simulink library "SUB_ECU_L4_MABX_HW_Interface"  (R2018a)
settings: Solver=VariableStepAuto  StartTime=0.0  StopTime=10.0  RelTol=1e-3
PostLoadFcn:
  | , if any(exist('dsrtsu_mdlpostloadfcn', 'file') == [2, 3, 6]), try dsrtsu_mdlpostloadfcn('Execute', bdroot); catch fprintf('Error in PostLoadFcn (dsrtsu_mdlpostloadfcn) for model "%s":\n %s\n', bdroot, lasterr); end, end,
undefined symbols (not defined in the file or in its folder): CANR_PROPB_REAX_3_13_CHANNEL_APV, CANR_PROPB_REAX_4_13_CHANNEL_APV, CANR_PROPB_XPR_1_50_CHANNEL_APV, ENUM_CAN_RX_T, ENUM_CAN_TX_T, ENUM_REAX_OPERATION_MODE_T, ENUM_SIGNAL_HEALTH_T, ENUM_XBR_CONTROL_MODE_T, ENUM_XBR_EBI_MODE_T, ENUM_XBR_PASS_THROUGH_ACTIVE_T, ENUM_XBR_PRIORITY_T, ENUM_XPR_INHIBIT_PARK_MANUAL_T, ENUM_XPR_INHIBIT_UNPARK_MANUAL_T, ENUM_XPR_PARK_MANUAL_T, ENUM_XPR_UNPARK_MANUAL_T, PROPB_REAX_1_E4_DES_POS_SIG_SRC_APV, PROPB_REAX_1_E4_DESIRED_OPMODE_APV, PROPB_REAX_1_E4_DESIRED_POSITION_APV, ptc_matlab_lib
libraries: PTC_MBDS_LIB x264, rtican x172, EmE_MBD_Blockset x39, simulink x34, $bdroot x16, rti1401lib_dio_type4 x8, simulink_need_slupdate x7, dsa_tcpip_lib x4, rti1401lib_adc_type4 x3, rtmapslib x3, rtitasklib x3
(part 33 of 51)

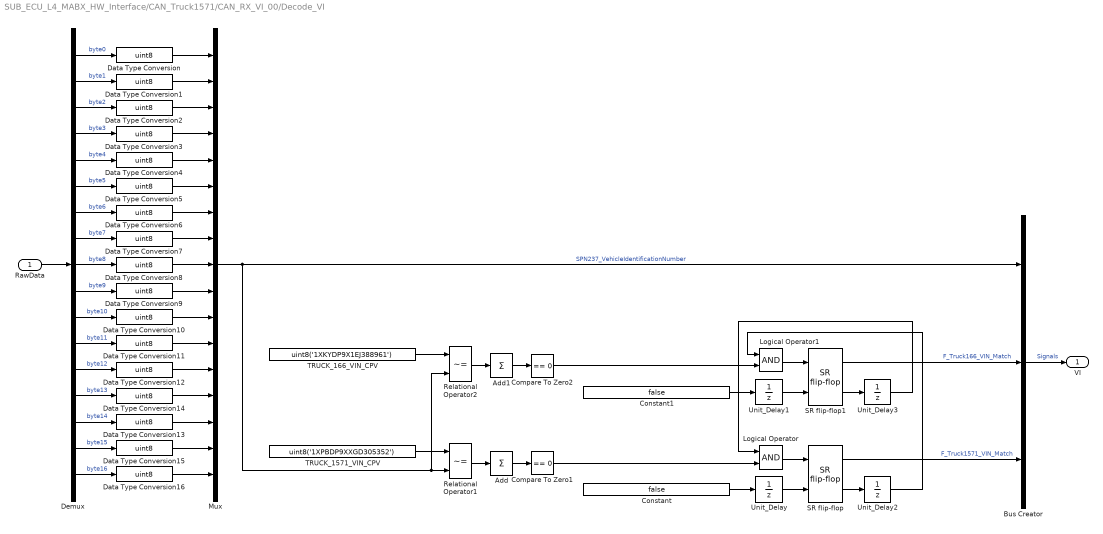
== system SUB_ECU_L4_MABX_HW_Interface/CAN_Truck1571/CAN_RX_VI_00/Decode_VI ==
  RawData : Inport  OutDataTypeStr=uint8  PortDimensions=17
  Add : Sum  Inputs=+  InputSameDT=on
  Add1 : Sum  Inputs=+  InputSameDT=on
  Bus Creator : BusCreator  Inputs=3
  Compare To Zero1 : simulink/Logic and Bit Operations/Compare To Zero  relop===  OutDataTypeStr=boolean
  Compare To Zero2 : simulink/Logic and Bit Operations/Compare To Zero  relop===  OutDataTypeStr=boolean
  Constant : Constant  Value=false
  Constant1 : Constant  Value=false
  Data Type Conversion{,1..16} (17 alike) : DataTypeConversion  OutDataTypeStr=uint8
  Demux : Demux  Outputs=17
  Logical Operator : Logic  OutDataTypeStr=boolean
  Logical Operator1 : Logic  OutDataTypeStr=boolean
  Mux : Mux  Inputs=17
  Relational Operator1 : RelationalOperator  Operator=~=  OutDataTypeStr=boolean  RndMeth=Nearest  InputSameDT=on
  Relational Operator2 : RelationalOperator  Operator=~=  OutDataTypeStr=boolean  RndMeth=Nearest  InputSameDT=on
  SR flip-flop : EmE_MBD_Blockset/Logic and Bit Operations/SR flip-flop
      settings: SourceProductName=PACCAR EmE MBD Blockset
  SR flip-flop1 : EmE_MBD_Blockset/Logic and Bit Operations/SR flip-flop
      settings: SourceProductName=PACCAR EmE MBD Blockset
  TRUCK_1571_VIN_CPV : Constant  Value=uint8('1XPBDP9XXGD305352')
  TRUCK_166_VIN_CPV : Constant  Value=uint8('1XKYDP9X1EJ388961')
  Unit_Delay{,1..3} (4 alike) : UnitDelay  InitialCondition=true  SampleTime=-1
      settings: AttributesFormatString=IC: %<vinit>
  VI : Outport
  wires:
  Unit_Delay3/1 -> Logical Operator/1
  Unit_Delay2/1 -> Logical Operator1/1
  SR flip-flop/2 -> Unit_Delay2/1
  Compare To Zero2/1 -> Logical Operator1/2
  Logical Operator1/1 -> SR flip-flop1/1
  Logical Operator/1 -> SR flip-flop/1
  SR flip-flop1/2 -> Unit_Delay3/1
  Constant1/1 -> Unit_Delay1/1
  Unit_Delay1/1 -> SR flip-flop1/2
  Compare To Zero1/1 -> Logical Operator/2
  Constant/1 -> Unit_Delay/1
  Unit_Delay/1 -> SR flip-flop/2
  Bus Creator/1 -> VI/1  "Signals"
  Demux/17 -> Data Type Conversion16/1  "byte16"
  Demux/16 -> Data Type Conversion15/1  "byte15"
  Demux/1 -> Data Type Conversion/1  "byte0"
  Demux/15 -> Data Type Conversion13/1  "byte14"
  Demux/14 -> Data Type Conversion14/1  "byte13"
  Demux/2 -> Data Type Conversion1/1  "byte1"
  Demux/3 -> Data Type Conversion2/1  "byte2"
  Demux/13 -> Data Type Conversion12/1  "byte12"
  Demux/4 -> Data Type Conversion3/1  "byte3"
  Demux/12 -> Data Type Conversion11/1  "byte11"
  Demux/5 -> Data Type Conversion4/1  "byte4"
  Demux/11 -> Data Type Conversion10/1  "byte10"
  Demux/10 -> Data Type Conversion9/1  "byte9"
  Demux/6 -> Data Type Conversion5/1  "byte5"
  Demux/7 -> Data Type Conversion6/1  "byte6"
  Demux/9 -> Data Type Conversion8/1  "byte8"
  Demux/8 -> Data Type Conversion7/1  "byte7"
  SR flip-flop1/1 -> Bus Creator/2  "F_Truck166_VIN_Match"
  SR flip-flop/1 -> Bus Creator/3  "F_Truck1571_VIN_Match"
  Add1/1 -> Compare To Zero2/1
  Relational Operator2/1 -> Add1/1
  TRUCK_1571_VIN_CPV/1 -> Relational Operator1/1
  TRUCK_166_VIN_CPV/1 -> Relational Operator2/1
  Add/1 -> Compare To Zero1/1
  Relational Operator1/1 -> Add/1
  Data Type Conversion14/1 -> Mux/14
  Data Type Conversion4/1 -> Mux/5
  Data Type Conversion9/1 -> Mux/10
  Data Type Conversion3/1 -> Mux/4
  Data Type Conversion2/1 -> Mux/3
  Data Type Conversion15/1 -> Mux/16
  Data Type Conversion8/1 -> Mux/9
  Data Type Conversion13/1 -> Mux/15
  Data Type Conversion12/1 -> Mux/13
  Data Type Conversion7/1 -> Mux/8
  Data Type Conversion11/1 -> Mux/12
  Data Type Conversion10/1 -> Mux/11
  Data Type Conversion6/1 -> Mux/7
  Data Type Conversion1/1 -> Mux/2
  Data Type Conversion/1 -> Mux/1
  Data Type Conversion5/1 -> Mux/6
  Data Type Conversion16/1 -> Mux/17
  Mux/1 -> Bus Creator/1, Relational Operator1/2, Relational Operator2/2  "SPN237_VehicleIdentificationNumber"
  RawData/1 -> Demux/1

== system SUB_ECU_L4_MABX_HW_Interface/CAN_Truck1571/Decode_PropB_REAX_3/decode_byte1 ==
  byte1 : Inport
  AND1 : PTC_MBDS_LIB/MBDS Standard Library/Basic Operations/Logic and Bit Operations/AND  BitwiseMode=on  Inputs=1  UseBitMask=on  BitMask=bin2dec('11110000')  OutDataTypeStr=uint8  PTC_MBDS_BlockVersion=5.41  PTC_BlockType=PTC_MBDS_AND
      settings: AttributesFormatString=bitwise  SourceProductName=PACCAR Technical Center MBDS Library
  AND2 : PTC_MBDS_LIB/MBDS Standard Library/Basic Operations/Logic and Bit Operations/AND  BitwiseMode=on  Inputs=1  UseBitMask=on  BitMask=bin2dec('00001111')  OutDataTypeStr=uint8  PTC_MBDS_BlockVersion=5.41  PTC_BlockType=PTC_MBDS_AND
      settings: AttributesFormatString=bitwise  SourceProductName=PACCAR Technical Center MBDS Library
  Bus Creator : BusCreator  Inputs=2
  "Shift_Arithmetic " : ArithShift  BitShiftNumber=4
  Out : Outport
  wires:
  Bus Creator/1 -> Out/1
  AND1/1 -> "Shift_Arithmetic "/1
  AND2/1 -> Bus Creator/1  "PropB_REAX_3_CurrentOperatingMode"
  byte1/1 -> AND2/1, AND1/1
  "Shift_Arithmetic "/1 -> Bus Creator/2  "PropB_REAX_3_ReqOperatingMode"

== system SUB_ECU_L4_MABX_HW_Interface/CAN_Truck1571/Decode_PropB_REAX_3/decode_byte2 ==
  byte2 : Inport
  Bus Creator : BusCreator  Inputs=1
  Out : Outport
  wires:
  Bus Creator/1 -> Out/1
  byte2/1 -> Bus Creator/1  "PropB_REAX_3_StatusErrMsg"

== system SUB_ECU_L4_MABX_HW_Interface/CAN_Truck1571/Decode_PropB_REAX_3/decode_byte3_byte4 ==
  byte3 : Inport
  byte4 : Inport  Port=2
  Bus Creator : BusCreator  Inputs=1
  Constant : Constant  Value=1/1024
  Data Type Conversion1 : DataTypeConversion  OutDataTypeStr=uint16  SaturateOnIntegerOverflow=on
  Data Type Conversion2 : DataTypeConversion  OutDataTypeStr=uint16  SaturateOnIntegerOverflow=on
  Data Type Conversion3 : DataTypeConversion  OutDataTypeStr=int16  ConvertRealWorld=Stored Integer (SI)
  Data Type Conversion4 : DataTypeConversion  SaturateOnIntegerOverflow=on
  OR : PTC_MBDS_LIB/MBDS Standard Library/Basic Operations/Logic and Bit Operations/OR  BitwiseMode=on  Inputs=2  UseBitMask=off  BitMask='A7'  OutDataTypeStr=uint16  PTC_MBDS_BlockVersion=5.41  PTC_BlockType=PTC_MBDS_OR
      settings: AttributesFormatString=bitwise  SourceProductName=PACCAR Technical Center MBDS Library
  Product : Product  Inputs=**  OutDataTypeStr=single  SaturateOnIntegerOverflow=on  InputSameDT=on
      settings: AttributesFormatString=Saturate: %<SaturateOnIntegerOverflow>
  Shift_Arithmetic 1 : ArithShift  BitShiftNumber=-8
  Out : Outport
  wires:
  Bus Creator/1 -> Out/1
  Data Type Conversion4/1 -> Product/1
  OR/1 -> Data Type Conversion3/1
  Shift_Arithmetic 1/1 -> OR/2
  Data Type Conversion1/1 -> OR/1
  Data Type Conversion2/1 -> Shift_Arithmetic 1/1
  byte4/1 -> Data Type Conversion2/1
  byte3/1 -> Data Type Conversion1/1
  Data Type Conversion3/1 -> Data Type Conversion4/1
  Constant/1 -> Product/2
  Product/1 -> Bus Creator/1  "PropB_REAX_3_HandwheelTorque"

== system SUB_ECU_L4_MABX_HW_Interface/CAN_Truck1571/Decode_PropB_REAX_3/decode_byte5_byte6 ==
  byte5 : Inport
  byte6 : Inport  Port=2
  Bus Creator : BusCreator  Inputs=1
  Constant1 : Constant  Value=1/1024
  Data Type Conversion1 : DataTypeConversion  SaturateOnIntegerOverflow=on
  Data Type Conversion4 : DataTypeConversion  OutDataTypeStr=uint16  SaturateOnIntegerOverflow=on
  Data Type Conversion5 : DataTypeConversion  OutDataTypeStr=uint16  SaturateOnIntegerOverflow=on
  Data Type Conversion6 : DataTypeConversion  OutDataTypeStr=int16  ConvertRealWorld=Stored Integer (SI)
  OR1 : PTC_MBDS_LIB/MBDS Standard Library/Basic Operations/Logic and Bit Operations/OR  BitwiseMode=on  Inputs=2  UseBitMask=off  BitMask='A7'  OutDataTypeStr=uint16  PTC_MBDS_BlockVersion=5.41  PTC_BlockType=PTC_MBDS_OR
      settings: AttributesFormatString=bitwise  SourceProductName=PACCAR Technical Center MBDS Library
  Product1 : Product  Inputs=**  OutDataTypeStr=single  SaturateOnIntegerOverflow=on  InputSameDT=on
      settings: AttributesFormatString=Saturate: %<SaturateOnIntegerOverflow>
  Shift_Arithmetic 2 : ArithShift  BitShiftNumber=-8
  Out : Outport
  wires:
  Bus Creator/1 -> Out/1
  Data Type Conversion1/1 -> Product1/1
  Product1/1 -> Bus Creator/1  "PropB_REAX_3_HandwheelVelocity"
  Constant1/1 -> Product1/2
  Data Type Conversion6/1 -> Data Type Conversion1/1
  OR1/1 -> Data Type Conversion6/1
  Data Type Conversion4/1 -> OR1/1
  Data Type Conversion5/1 -> Shift_Arithmetic 2/1
  Shift_Arithmetic 2/1 -> OR1/2
  byte6/1 -> Data Type Conversion5/1
  byte5/1 -> Data Type Conversion4/1

== system SUB_ECU_L4_MABX_HW_Interface/CAN_Truck1571/Decode_PropB_REAX_3/decode_byte7_byte8 ==
  byte7 : Inport
  byte8 : Inport  Port=2
  Bus Creator : BusCreator  Inputs=1
  Constant2 : Constant  Value=360/8192
  Data Type Conversion1 : DataTypeConversion  SaturateOnIntegerOverflow=on
  Data Type Conversion7 : DataTypeConversion  OutDataTypeStr=uint16  SaturateOnIntegerOverflow=on
  Data Type Conversion8 : DataTypeConversion  OutDataTypeStr=uint16  SaturateOnIntegerOverflow=on
  Data Type Conversion9 : DataTypeConversion  OutDataTypeStr=int16  ConvertRealWorld=Stored Integer (SI)
  OR2 : PTC_MBDS_LIB/MBDS Standard Library/Basic Operations/Logic and Bit Operations/OR  BitwiseMode=on  Inputs=2  UseBitMask=off  BitMask='A7'  OutDataTypeStr=uint16  PTC_MBDS_BlockVersion=5.41  PTC_BlockType=PTC_MBDS_OR
      settings: AttributesFormatString=bitwise  SourceProductName=PACCAR Technical Center MBDS Library
  Product2 : Product  Inputs=**  OutDataTypeStr=single  SaturateOnIntegerOverflow=on  InputSameDT=on
      settings: AttributesFormatString=Saturate: %<SaturateOnIntegerOverflow>
  Shift_Arithmetic 3 : ArithShift  BitShiftNumber=-8
  Out : Outport
  wires:
  Bus Creator/1 -> Out/1
  Data Type Conversion1/1 -> Product2/1
  Data Type Conversion9/1 -> Data Type Conversion1/1
  Constant2/1 -> Product2/2
  OR2/1 -> Data Type Conversion9/1
  Shift_Arithmetic 3/1 -> OR2/2
  Data Type Conversion7/1 -> OR2/1
  Data Type Conversion8/1 -> Shift_Arithmetic 3/1
  byte7/1 -> Data Type Conversion7/1
  Product2/1 -> Bus Creator/1  "PropB_REAX_3_PullCompensation"
  byte8/1 -> Data Type Conversion8/1

== system SUB_ECU_L4_MABX_HW_Interface/CAN_Truck1571/Decode_PropB_REAX_4/decode_byte1 ==
  byte1 : Inport
  AND : PTC_MBDS_LIB/MBDS Standard Library/Basic Operations/Logic and Bit Operations/AND  BitwiseMode=on  Inputs=1  UseBitMask=on  BitMask=bin2dec('00000001')  OutDataTypeStr=boolean  PTC_MBDS_BlockVersion=5.41  PTC_BlockType=PTC_MBDS_AND
      settings: AttributesFormatString=bitwise  SourceProductName=PACCAR Technical Center MBDS Library
  AND1 : PTC_MBDS_LIB/MBDS Standard Library/Basic Operations/Logic and Bit Operations/AND  BitwiseMode=on  Inputs=1  UseBitMask=on  BitMask=bin2dec('00000010')  OutDataTypeStr=uint8  PTC_MBDS_BlockVersion=5.41  PTC_BlockType=PTC_MBDS_AND
      settings: AttributesFormatString=bitwise  SourceProductName=PACCAR Technical Center MBDS Library
  AND2 : PTC_MBDS_LIB/MBDS Standard Library/Basic Operations/Logic and Bit Operations/AND  BitwiseMode=on  Inputs=1  UseBitMask=on  BitMask=bin2dec('00000100')  OutDataTypeStr=uint8  PTC_MBDS_BlockVersion=5.41  PTC_BlockType=PTC_MBDS_AND
      settings: AttributesFormatString=bitwise  SourceProductName=PACCAR Technical Center MBDS Library
  Bus Creator : BusCreator  Inputs=3
  Data Type Conversion : DataTypeConversion  OutDataTypeStr=boolean  SaturateOnIntegerOverflow=on
  Data Type Conversion1 : DataTypeConversion  OutDataTypeStr=boolean  SaturateOnIntegerOverflow=on
  "Shift_Arithmetic " : ArithShift  BitShiftNumber=1
  Shift_Arithmetic 1 : ArithShift  BitShiftNumber=2
  Out : Outport
  wires:
  Data Type Conversion1/1 -> Bus Creator/3  "PropB_REAX_4_DriverControlledEffortsEnabled"
  Data Type Conversion/1 -> Bus Creator/2  "PropB_REAX_4_PositionIndexValid"
  Bus Creator/1 -> Out/1
  Shift_Arithmetic 1/1 -> Data Type Conversion1/1
  "Shift_Arithmetic "/1 -> Data Type Conversion/1
  AND1/1 -> "Shift_Arithmetic "/1
  byte1/1 -> AND/1, AND1/1, AND2/1
  AND2/1 -> Shift_Arithmetic 1/1
  AND/1 -> Bus Creator/1  "PropB_REAX_4_AbsSteeringPosValid"

== system SUB_ECU_L4_MABX_HW_Interface/CAN_Truck1571/Decode_PropB_REAX_4/decode_byte2 ==
  byte2 : Inport
  Bus Creator : BusCreator  Inputs=1
  SignalConversion : SignalConversion  ConversionOutput=Contiguous copy  OverrideOpt=off
  Out : Outport
  wires:
  Bus Creator/1 -> Out/1
  SignalConversion/1 -> Bus Creator/1  "PropB_REAX_4_ControlOperatingMode"
  byte2/1 -> SignalConversion/1

== system SUB_ECU_L4_MABX_HW_Interface/CAN_Truck1571/Decode_PropB_REAX_4/decode_byte3 ==
  byte3 : Inport
  Bus Creator : BusCreator  Inputs=1
  SignalConversion : SignalConversion  ConversionOutput=Contiguous copy  OverrideOpt=off
  Out : Outport
  wires:
  Bus Creator/1 -> Out/1
  SignalConversion/1 -> Bus Creator/1  "PropB_REAX_4_SystemMode"
  byte3/1 -> SignalConversion/1

== system SUB_ECU_L4_MABX_HW_Interface/CAN_Truck1571/Decode_PropB_REAX_4/decode_byte5 ==
  byte5 : Inport
  Bus Creator : BusCreator  Inputs=1
  Data Type Conversion4 : DataTypeConversion  OutDataTypeStr=int8  ConvertRealWorld=Stored Integer (SI)
  Data Type Conversion5 : DataTypeConversion  OutDataTypeStr=double  SaturateOnIntegerOverflow=on
  Out : Outport
  wires:
  Bus Creator/1 -> Out/1
  Data Type Conversion5/1 -> Bus Creator/1  "PropB_REAX_4_PercHandwheelTorque"
  Data Type Conversion4/1 -> Data Type Conversion5/1
  byte5/1 -> Data Type Conversion4/1

== system SUB_ECU_L4_MABX_HW_Interface/CAN_Truck1571/Decode_PropB_REAX_4/decode_byte6_byte7 ==
  byte6 : Inport
  byte7 : Inport  Port=2
  Bus Creator : BusCreator  Inputs=1
  Data Type Conversion6 : DataTypeConversion  OutDataTypeStr=uint16  SaturateOnIntegerOverflow=on
  Data Type Conversion7 : DataTypeConversion  OutDataTypeStr=uint16  SaturateOnIntegerOverflow=on
  Data Type Conversion8 : DataTypeConversion  OutDataTypeStr=int16  ConvertRealWorld=Stored Integer (SI)
  Data Type Conversion9 : DataTypeConversion  OutDataTypeStr=double  SaturateOnIntegerOverflow=on
  OR : PTC_MBDS_LIB/MBDS Standard Library/Basic Operations/Logic and Bit Operations/OR  BitwiseMode=on  Inputs=2  UseBitMask=off  BitMask='A7'  OutDataTypeStr=uint16  PTC_MBDS_BlockVersion=5.41  PTC_BlockType=PTC_MBDS_OR
      settings: AttributesFormatString=bitwise  SourceProductName=PACCAR Technical Center MBDS Library
  Shift_Arithmetic 2 : ArithShift  BitShiftNumber=-8
  Out : Outport
  wires:
  Bus Creator/1 -> Out/1
  OR/1 -> Data Type Conversion8/1
  Data Type Conversion8/1 -> Data Type Conversion9/1
  Shift_Arithmetic 2/1 -> OR/2
  Data Type Conversion7/1 -> Shift_Arithmetic 2/1
  Data Type Conversion6/1 -> OR/1
  byte7/1 -> Data Type Conversion7/1
  byte6/1 -> Data Type Conversion6/1
  Data Type Conversion9/1 -> Bus Creator/1  "PropB_REAX_4_AbsSteeringAngle"

== system SUB_ECU_L4_MABX_HW_Interface/CAN_Truck1571/Decode_PropB_REAX_4/decode_byte8 ==
  byte8 : Inport
  Bus Creator : BusCreator  Inputs=1
  Data Type Conversion10 : DataTypeConversion  OutDataTypeStr=int8  ConvertRealWorld=Stored Integer (SI)
  Data Type Conversion11 : DataTypeConversion  OutDataTypeStr=double  SaturateOnIntegerOverflow=on
  Out : Outport
  wires:
  Bus Creator/1 -> Out/1
  byte8/1 -> Data Type Conversion10/1
  Data Type Conversion10/1 -> Data Type Conversion11/1
  Data Type Conversion11/1 -> Bus Creator/1  "PropB_REAX_4_PercMotorTorque"

== system SUB_ECU_L4_MABX_HW_Interface/CAN_Truck166/CAN1_RX_TPCM_FF_00/RX_CAN_1 ==
  Enable : Inport
  Bus Creator3 : BusCreator  Inputs=4
  CAN_TYPE1_RX_M1_C1 : rtican/RTICAN Receive (RX)   Reserved1=[]  Reserved2=[]  Reserved3=[]  Reserved4=[]  SfcnMessage=[]  Msg_Struct=[]  BoardTypeNo=[]  BoardNo=[]  ChannelNo=[]  Parameters=[]  DialogFcn=[]  UnitName=[]  Revision=[]  UnitValues=[]  DSProperties=struct('RTI',struct('Version',uint32(5),'BlockType',struct('isSLSource',uint8(1),'isSLSink',uint8(1),'isHWSource',uint8(0),'isHWSink',uint8(0),'isSetup',uint8(0),'isInline',uint8(1),'isNonInline',uint8(0),'isInterrupt',uint8(0),'isChannelwise',uint8(0)),'IOBoardType','RTICAN','UnitType','MESSAGE','Identifier','RX','DialogType','MSVC','BlockSet','RTICAN','SlaveProcessor','CAN'))  RTIBlockInterface=struct('OutputPortsWidth',int32([1 1 1 1 1 1 1 1 1 1 1]),'OutputPortsActive',ones(1,11),'OutputPortsName',{{'byte1','byte2','byte3','byte4','byte5','byte6','byte7','byte8',['RX status'],['RX time'],['RX delta time']}},'OutputPortsDataType',{{'SS_DOUBLE','SS_DOUBLE','SS_DOUBLE','SS_DOUBLE','SS_DOUBLE','SS_DOUBLE','SS_DOUBLE','SS_DOUBLE','SS_DOUBLE','SS_DOUBLE','SS_DOUBLE'}},'OutputPortsLabel',{{'byte1','byte2','byte3','byte4','byte5','byte6','byte7','byte8','','',''}},'OutputPortsLabelMode','ON','InputPortsWidth',int32(0),'InputPortsActive',0,'DialogFcn','rtican_message_interface_gui','BlockDisplay',{{'','center'}},'IconTransparency','on','ParameterTunableNames',{{}},'InitLevel',3,'BlockName',struct('Token',{{'CAN_TYPE','_RX_M','_C'}},'BlockParam',{{'BoardTypeNo','BoardNo','ChannelNo'}}),'SampleTime',{{-1}},'TriggerPort',{{'none'}},'EnablePort',{{'yes'}})  RTIBlockParameters=struct('BoardTypeNo',{{1,'OFF',[]}},'BoardNo',{{1,'ON',[1 16]}},'ChannelNo',{{1,'ON',[1 2]}},'Parameters',{{struct('DataFileSupport',struct('DataFileSelectedMaster',1,'DataFileSelectedLocal',0,'DataFileName','c:\data\svn\ptc_autonomous_truck_secure\trunk\candb\selfdrivingtruck.dbc|','DataFileDate',{{{['04-Nov-2016 10:11:27']}}},'SelectedFile',['<no file selected>']),'Options',struct('StatusSelected',1,'TimeSelected',1,'DeltaTimeSelected',1,'BytePortSelected',0,'MessageLengthSelected',0,'TriggerPort',struct('Selected',0,'TriggerType',0),'UserCoding',struct('Selected',0,'InterfaceFile','UserDecodingFile','FcnName','UserDecodeFcn','InportSelected',0,'InportWidth',1,'OutportSelected',0,'OutportWidth',1),'EnablePortSelected',1,'SignalOnPortnameSelected',1,'UseRXService',1),'Message',struct('MsgOnBlocknameSelected',0,'MsgName','TPCM_FF_00','MsgIdFormat',1,'MsgId',485293824,'MsgLength',8,'NumSignals',8,'SampleTime',-1,'Signal',struct('SgnName',{'byte1','byte2','byte3','byte4','byte5','byte6','byte7','byte8'},'SgnStartBit',{0,8,16,24,32,40,48,56},'SgnLength',{8,8,8,8,8,8,8,8},'SgnType',{0,0,0,0,0,0,0,0},'ModeValue',{-1,-1,-1,-1,-1,-1,-1,-1},'DataType',{0,0,0,0,0,0,0,0},'ByteLayout',{0,0,0,0,0,0,0,0},'Factor',{1,1,1,1,1,1,1,1},'Offset',{0,0,0,0,0,0,0,0},'SgnComment',{{''},{''},{''},{''},{''},{''},{''},{''}},'SgnUnit',{'','','','','','','',''},'Min',{0,0,0,0,0,0,0,0},'Max',{0,0,0,0,0,0,0,0},'SLDataType',{'SS_DOUBLE','SS_DOUBLE','SS_DOUBLE','SS_DOUBLE','SS_DOUBLE','SS_DOUBLE','SS_DOUBLE','SS_DOUBLE'}),'MsgIdNumFormat',1,'MsgComment',{{'TPCM_FF_00'}}),'Version',1.2,'general',struct('isFromLib',0)),'OFF',[]}},'GroupId',{{struct('Group',{{'RTICAN'}},'No',1,'Behavior',{{'NAMECHANGE'}},'BlockType',{{'SINK'}},'NameChangeFlag',0),'OFF',[]}},'SFcnRTICANMessage',{{struct('MsgType','RX','SFcnPortType','Scalar','MsgName','TPCM_FF_00','MsgIdFormat','XTD','MsgId',485293824,'MsgLength',8,'NumSignals',8,'SampleTime',-1,'Signal',struct('SgnName',{'byte1','byte2','byte3','byte4','byte5','byte6','byte7','byte8'},'SgnStartBit',{0,8,16,24,32,40,48,56},'SgnLength',{8,8,8,8,8,8,8,8},'SgnType',{'standard','standard','standard','standard','standard','standard','standard','standard'},'ModeValue',{-1,-1,-1,-1,-1,-1,-1,-1},'DataType',{['unsigned int'],['unsigned int'],['unsigned int'],['unsigned int'],['unsigned int'],['unsigned int'],['unsigned int'],['unsigned int']},'ByteLayout',{['little endian'],['little endian'],['little endian'],['little endian'],['little endian'],['little endian'],['little endian'],['little endian']},'Factor',{1,1,1,1,1,1,1,1},'Offset',{0,0,0,0,0,0,0,0},'SLDataType',{'SS_DOUBLE','SS_DOUBLE','SS_DOUBLE','SS_DOUBLE','SS_DOUBLE','SS_DOUBLE','SS_DOUBLE','SS_DOUBLE'}),'StatusSelected','yes','TimeSelected','yes','DeltaTimeSelected','yes','BytePortSelected','no','MessageLengthSelected','no','TriggerPort',struct('Selected','no','TriggerType',0),'UserCoding',struct('Selected','no','InterfaceFile','UserDecodingFile','FcnName','UserDecodeFcn','InportSelected','no','InportWidth',1,'OutportSelected','no','OutportWidth',1),'EnablePortSelected','yes','UseRXService','yes','BoardType','DS1','BoardNo',1,'ControllerNo',1),'OFF',[]}},'TLCFileName',{{'rtican_rx_message','OFF',[]}})  RTISFcnParameters=struct('SFcnRTICANMessage','struct','TLCFileName','char')  RTIBlockParaDefault=struct('BoardTypeNo',4302,'BoardNo',1,'ChannelNo',1,'Parameters',struct('DataFileSupport',struct('DataFileSelectedMaster',0,'DataFileSelectedLocal',0,'DataFileName','','DataFileDate','','SelectedFile',['<no file selected>']),'Options',struct('StatusSelected',1,'TimeSelected',1,'DeltaTimeSelected',1,'BytePortSelected',0,'MessageLengthSelected',0,'TriggerPort',struct('Selected',0,'TriggerType','rising'),'UserCoding',struct('Selected',0,'InterfaceFile','UserDecodingFile','FcnName','UserDecodeFcn','InportSelected',0,'InportWidth',1,'OutportSelected',0,'OutportWidth',1),'EnablePortSelected',0,'SignalOnPortnameSelected',1,'UseRXService',0),'Message',struct('MsgOnBlocknameSelected',0,'MsgName',['RX Message'],'MsgIdFormat',0,'MsgId',100,'MsgLength',8,'NumSignals',1,'SampleTime',-1,'Signal',struct('SgnName',['RX signal'],'SgnStartBit',0,'SgnLength',8,'SgnType',0,'ModeValue',-1,'DataType',0,'SLDataType','SS_DOUBLE','ByteLayout',0,'Factor',1,'Offset',0,'Min',0,'Max',255,'SgnComment',{{}},'SgnUnit',''),'MsgIdNumFormat',0,'MsgComment',{{''}}),'Version',1.2,'general',struct('isFromLib',1)),'GroupId',struct('Group',{{'RTICAN'}},'No',1,'Behavior',{{'NAMECHANGE'}},'BlockType',{{'SINK'}},'NameChangeFlag',0),'SFcnRTICANMessage',struct('MsgType','RX','MsgName',['RX Message'],'MsgIdFormat','STD','MsgId',100,'MsgLength',8,'NumSignals',1,'SampleTime',-1,'Signal',struct('SgnName',['RX signal'],'SgnStartBit',0,'SgnLength',8,'SgnType','standard','ModeValue',-1,'DataType',['unsigned int'],'ByteLayout',['little endian'],'SLDataType','SS_DOUBLE','Factor',1,'Offset',0),'StatusSelected','yes','TimeSelected','yes','DeltaTimeSelected','yes','BytePortSelected','no','MessageLengthSelected','no','EnablePortSelected','no','UserCoding',struct('Selected','no','InterfaceFile','UserDecodingFile','FcnName','UserDecodeFcn','InportSelected','no','InportWidth',1,'OutportSelected','no','OutportWidth',1),'TriggerPort',struct('Selected','no','TriggerType','rising'),'UseRXService','no','BoardType','DS4302','BoardNo',1,'ControllerNo',1,'SFcnPortType','Scalar'),'TLCFileName','rtican_rx_message')
      settings: AttributesFormatString=Group Id: RTICAN1\n  SourceProductName=dSPACE RTI CAN Blockset
  Data Type Conversion{,1..7} (8 alike) : DataTypeConversion  OutDataTypeStr=uint8  SaturateOnIntegerOverflow=on
  Data Type Conversion10 : DataTypeConversion  OutDataTypeStr=double  SaturateOnIntegerOverflow=on
  Data Type Conversion8 : DataTypeConversion  OutDataTypeStr=boolean  SaturateOnIntegerOverflow=on
  Data Type Conversion9 : DataTypeConversion  OutDataTypeStr=double  SaturateOnIntegerOverflow=on
  Mux : Mux  Inputs=8
  TPCM_FF_00 : Outport
  wires:
  Data Type Conversion9/1 -> Bus Creator3/3  "RX_time"
  Data Type Conversion10/1 -> Bus Creator3/4  "RX_delta_time"
  Data Type Conversion8/1 -> Bus Creator3/2  "RX_status"
  Bus Creator3/1 -> TPCM_FF_00/1  "TPCM_FF_00"
  CAN_TYPE1_RX_M1_C1/1 -> Data Type Conversion/1  "byte1"
  CAN_TYPE1_RX_M1_C1/3 -> Data Type Conversion2/1  "byte3"
  CAN_TYPE1_RX_M1_C1/4 -> Data Type Conversion3/1  "byte4"
  CAN_TYPE1_RX_M1_C1/2 -> Data Type Conversion1/1  "byte2"
  CAN_TYPE1_RX_M1_C1/6 -> Data Type Conversion5/1  "byte6"
  CAN_TYPE1_RX_M1_C1/5 -> Data Type Conversion4/1  "byte5"
  CAN_TYPE1_RX_M1_C1/8 -> Data Type Conversion7/1  "byte8"
  CAN_TYPE1_RX_M1_C1/7 -> Data Type Conversion6/1  "byte7"
  Data Type Conversion3/1 -> Mux/4
  Data Type Conversion4/1 -> Mux/5
  Data Type Conversion2/1 -> Mux/3
  Data Type Conversion5/1 -> Mux/6
  Data Type Conversion1/1 -> Mux/2
  Data Type Conversion6/1 -> Mux/7
  Data Type Conversion/1 -> Mux/1
  Data Type Conversion7/1 -> Mux/8
  Mux/1 -> Bus Creator3/1  "RawData"
  CAN_TYPE1_RX_M1_C1/11 -> Data Type Conversion10/1
  CAN_TYPE1_RX_M1_C1/10 -> Data Type Conversion9/1
  CAN_TYPE1_RX_M1_C1/9 -> Data Type Conversion8/1
  Enable/1 -> CAN_TYPE1_RX_M1_C1/Enable

== system SUB_ECU_L4_MABX_HW_Interface/CAN_Truck166/CAN1_RX_TPCM_FF_00/SelectChannel ==
  In1 : Inport
  Constant : Constant  Value=ENUM_CAN_RX_T.RX_CAN_1
  Constant1 : Constant  Value=ENUM_CAN_RX_T.RX_CAN_2
  Constant2 : Constant  Value=ENUM_CAN_RX_T.RX_CAN_3
  Constant3 : Constant  Value=ENUM_CAN_RX_T.RX_CAN_4
  Constant4 : Constant  Value=ENUM_CAN_RX_T.RX_CAN_5
  Constant5 : Constant  Value=ENUM_CAN_RX_T.RX_CAN_6
  EQ{,1..5} (6 alike) : PTC_MBDS_LIB/MBDS Standard Library/Basic Operations/Logic and Bit Operations/EQ  InputSameDT=on  PTC_MBDS_BlockVersion=5.41  PTC_BlockType=PTC_MBDS_EQ
      settings: SourceProductName=PACCAR Technical Center MBDS Library
  CAN1 : Outport
  CAN2 : Outport  Port=2
  CAN3 : Outport  Port=3
  CAN4 : Outport  Port=4
  CAN5 : Outport  Port=5
  CAN6 : Outport  Port=6
  wires:
  In1/1 -> EQ5/1, EQ4/1, EQ3/1, EQ2/1, EQ1/1, EQ/1
  Constant/1 -> EQ/2
  EQ/1 -> CAN1/1
  Constant1/1 -> EQ1/2
  Constant2/1 -> EQ2/2
  Constant3/1 -> EQ3/2
  Constant4/1 -> EQ4/2
  Constant5/1 -> EQ5/2
  EQ1/1 -> CAN2/1
  EQ2/1 -> CAN3/1
  EQ3/1 -> CAN4/1
  EQ4/1 -> CAN5/1
  EQ5/1 -> CAN6/1

== system SUB_ECU_L4_MABX_HW_Interface/CAN_Truck166/CAN1_RX_TPDT_FF_00/RX_CAN_1 ==
  Enable : Inport
  Bus Creator3 : BusCreator  Inputs=4
  CAN_TYPE1_RX_M1_C1 : rtican/RTICAN Receive (RX)   Reserved1=[]  Reserved2=[]  Reserved3=[]  Reserved4=[]  SfcnMessage=[]  Msg_Struct=[]  BoardTypeNo=[]  BoardNo=[]  ChannelNo=[]  Parameters=[]  DialogFcn=[]  UnitName=[]  Revision=[]  UnitValues=[]  DSProperties=struct('RTI',struct('Version',uint32(5),'BlockType',struct('isSLSource',uint8(1),'isSLSink',uint8(1),'isHWSource',uint8(0),'isHWSink',uint8(0),'isSetup',uint8(0),'isInline',uint8(1),'isNonInline',uint8(0),'isInterrupt',uint8(0),'isChannelwise',uint8(0)),'IOBoardType','RTICAN','UnitType','MESSAGE','Identifier','RX','DialogType','MSVC','BlockSet','RTICAN','SlaveProcessor','CAN'))  RTIBlockInterface=struct('OutputPortsWidth',int32([1 1 1 1 1 1 1 1 1 1 1]),'OutputPortsActive',ones(1,11),'OutputPortsName',{{'byte1','byte2','byte3','byte4','byte5','byte6','byte7','byte8',['RX status'],['RX time'],['RX delta time']}},'OutputPortsDataType',{{'SS_DOUBLE','SS_DOUBLE','SS_DOUBLE','SS_DOUBLE','SS_DOUBLE','SS_DOUBLE','SS_DOUBLE','SS_DOUBLE','SS_DOUBLE','SS_DOUBLE','SS_DOUBLE'}},'OutputPortsLabel',{{'byte1','byte2','byte3','byte4','byte5','byte6','byte7','byte8','','',''}},'OutputPortsLabelMode','ON','InputPortsWidth',int32(0),'InputPortsActive',0,'DialogFcn','rtican_message_interface_gui','BlockDisplay',{{'','center'}},'IconTransparency','on','ParameterTunableNames',{{}},'InitLevel',3,'BlockName',struct('Token',{{'CAN_TYPE','_RX_M','_C'}},'BlockParam',{{'BoardTypeNo','BoardNo','ChannelNo'}}),'SampleTime',{{-1}},'TriggerPort',{{'none'}},'EnablePort',{{'yes'}})  RTIBlockParameters=struct('BoardTypeNo',{{1,'OFF',[]}},'BoardNo',{{1,'ON',[1 16]}},'ChannelNo',{{1,'ON',[1 2]}},'Parameters',{{struct('DataFileSupport',struct('DataFileSelectedMaster',1,'DataFileSelectedLocal',0,'DataFileName','c:\data\svn\ptc_autonomous_truck_secure\trunk\candb\selfdrivingtruck.dbc|','DataFileDate',{{{['04-Nov-2016 10:11:27']}}},'SelectedFile',['<no file selected>']),'Options',struct('StatusSelected',1,'TimeSelected',1,'DeltaTimeSelected',1,'BytePortSelected',0,'MessageLengthSelected',0,'TriggerPort',struct('Selected',0,'TriggerType',0),'UserCoding',struct('Selected',0,'InterfaceFile','UserDecodingFile','FcnName','UserDecodeFcn','InportSelected',0,'InportWidth',1,'OutportSelected',0,'OutportWidth',1),'EnablePortSelected',1,'SignalOnPortnameSelected',1,'UseRXService',1),'Message',struct('MsgOnBlocknameSelected',0,'MsgName','TPDT_FF_00','MsgIdFormat',1,'MsgId',485228288,'MsgLength',8,'NumSignals',8,'SampleTime',-1,'Signal',struct('SgnName',{'byte1','byte2','byte3','byte4','byte5','byte6','byte7','byte8'},'SgnStartBit',{0,8,16,24,32,40,48,56},'SgnLength',{8,8,8,8,8,8,8,8},'SgnType',{0,0,0,0,0,0,0,0},'ModeValue',{-1,-1,-1,-1,-1,-1,-1,-1},'DataType',{0,0,0,0,0,0,0,0},'ByteLayout',{0,0,0,0,0,0,0,0},'Factor',{1,1,1,1,1,1,1,1},'Offset',{0,0,0,0,0,0,0,0},'SgnComment',{{''},{''},{''},{''},{''},{''},{''},{''}},'SgnUnit',{'','','','','','','',''},'Min',{0,0,0,0,0,0,0,0},'Max',{0,0,0,0,0,0,0,0},'SLDataType',{'SS_DOUBLE','SS_DOUBLE','SS_DOUBLE','SS_DOUBLE','SS_DOUBLE','SS_DOUBLE','SS_DOUBLE','SS_DOUBLE'}),'MsgIdNumFormat',1,'MsgComment',{{'TPDT_FF_00'}}),'Version',1.2,'general',struct('isFromLib',0)),'OFF',[]}},'GroupId',{{struct('Group',{{'RTICAN'}},'No',1,'Behavior',{{'NAMECHANGE'}},'BlockType',{{'SINK'}},'NameChangeFlag',0),'OFF',[]}},'SFcnRTICANMessage',{{struct('MsgType','RX','SFcnPortType','Scalar','MsgName','TPDT_FF_00','MsgIdFormat','XTD','MsgId',485228288,'MsgLength',8,'NumSignals',8,'SampleTime',-1,'Signal',struct('SgnName',{'byte1','byte2','byte3','byte4','byte5','byte6','byte7','byte8'},'SgnStartBit',{0,8,16,24,32,40,48,56},'SgnLength',{8,8,8,8,8,8,8,8},'SgnType',{'standard','standard','standard','standard','standard','standard','standard','standard'},'ModeValue',{-1,-1,-1,-1,-1,-1,-1,-1},'DataType',{['unsigned int'],['unsigned int'],['unsigned int'],['unsigned int'],['unsigned int'],['unsigned int'],['unsigned int'],['unsigned int']},'ByteLayout',{['little endian'],['little endian'],['little endian'],['little endian'],['little endian'],['little endian'],['little endian'],['little endian']},'Factor',{1,1,1,1,1,1,1,1},'Offset',{0,0,0,0,0,0,0,0},'SLDataType',{'SS_DOUBLE','SS_DOUBLE','SS_DOUBLE','SS_DOUBLE','SS_DOUBLE','SS_DOUBLE','SS_DOUBLE','SS_DOUBLE'}),'StatusSelected','yes','TimeSelected','yes','DeltaTimeSelected','yes','BytePortSelected','no','MessageLengthSelected','no','TriggerPort',struct('Selected','no','TriggerType',0),'UserCoding',struct('Selected','no','InterfaceFile','UserDecodingFile','FcnName','UserDecodeFcn','InportSelected','no','InportWidth',1,'OutportSelected','no','OutportWidth',1),'EnablePortSelected','yes','UseRXService','yes','BoardType','DS1','BoardNo',1,'ControllerNo',1),'OFF',[]}},'TLCFileName',{{'rtican_rx_message','OFF',[]}})  RTISFcnParameters=struct('SFcnRTICANMessage','struct','TLCFileName','char')  RTIBlockParaDefault=struct('BoardTypeNo',4302,'BoardNo',1,'ChannelNo',1,'Parameters',struct('DataFileSupport',struct('DataFileSelectedMaster',0,'DataFileSelectedLocal',0,'DataFileName','','DataFileDate','','SelectedFile',['<no file selected>']),'Options',struct('StatusSelected',1,'TimeSelected',1,'DeltaTimeSelected',1,'BytePortSelected',0,'MessageLengthSelected',0,'TriggerPort',struct('Selected',0,'TriggerType','rising'),'UserCoding',struct('Selected',0,'InterfaceFile','UserDecodingFile','FcnName','UserDecodeFcn','InportSelected',0,'InportWidth',1,'OutportSelected',0,'OutportWidth',1),'EnablePortSelected',0,'SignalOnPortnameSelected',1,'UseRXService',0),'Message',struct('MsgOnBlocknameSelected',0,'MsgName',['RX Message'],'MsgIdFormat',0,'MsgId',100,'MsgLength',8,'NumSignals',1,'SampleTime',-1,'Signal',struct('SgnName',['RX signal'],'SgnStartBit',0,'SgnLength',8,'SgnType',0,'ModeValue',-1,'DataType',0,'SLDataType','SS_DOUBLE','ByteLayout',0,'Factor',1,'Offset',0,'Min',0,'Max',255,'SgnComment',{{}},'SgnUnit',''),'MsgIdNumFormat',0,'MsgComment',{{''}}),'Version',1.2,'general',struct('isFromLib',1)),'GroupId',struct('Group',{{'RTICAN'}},'No',1,'Behavior',{{'NAMECHANGE'}},'BlockType',{{'SINK'}},'NameChangeFlag',0),'SFcnRTICANMessage',struct('MsgType','RX','MsgName',['RX Message'],'MsgIdFormat','STD','MsgId',100,'MsgLength',8,'NumSignals',1,'SampleTime',-1,'Signal',struct('SgnName',['RX signal'],'SgnStartBit',0,'SgnLength',8,'SgnType','standard','ModeValue',-1,'DataType',['unsigned int'],'ByteLayout',['little endian'],'SLDataType','SS_DOUBLE','Factor',1,'Offset',0),'StatusSelected','yes','TimeSelected','yes','DeltaTimeSelected','yes','BytePortSelected','no','MessageLengthSelected','no','EnablePortSelected','no','UserCoding',struct('Selected','no','InterfaceFile','UserDecodingFile','FcnName','UserDecodeFcn','InportSelected','no','InportWidth',1,'OutportSelected','no','OutportWidth',1),'TriggerPort',struct('Selected','no','TriggerType','rising'),'UseRXService','no','BoardType','DS4302','BoardNo',1,'ControllerNo',1,'SFcnPortType','Scalar'),'TLCFileName','rtican_rx_message')
      settings: AttributesFormatString=Group Id: RTICAN1\n  SourceProductName=dSPACE RTI CAN Blockset
  Data Type Conversion{,1..7} (8 alike) : DataTypeConversion  OutDataTypeStr=uint8  SaturateOnIntegerOverflow=on
  Data Type Conversion10 : DataTypeConversion  OutDataTypeStr=double  SaturateOnIntegerOverflow=on
  Data Type Conversion8 : DataTypeConversion  OutDataTypeStr=boolean  SaturateOnIntegerOverflow=on
  Data Type Conversion9 : DataTypeConversion  OutDataTypeStr=double  SaturateOnIntegerOverflow=on
  Mux : Mux  Inputs=8
  TPDT_FF_00 : Outport
  wires:
  Data Type Conversion9/1 -> Bus Creator3/3  "RX_time"
  Data Type Conversion10/1 -> Bus Creator3/4  "RX_delta_time"
  Data Type Conversion8/1 -> Bus Creator3/2  "RX_status"
  Enable/1 -> CAN_TYPE1_RX_M1_C1/Enable
  CAN_TYPE1_RX_M1_C1/9 -> Data Type Conversion8/1
  CAN_TYPE1_RX_M1_C1/10 -> Data Type Conversion9/1
  CAN_TYPE1_RX_M1_C1/11 -> Data Type Conversion10/1
  Mux/1 -> Bus Creator3/1  "RawData"
  Data Type Conversion7/1 -> Mux/8
  Data Type Conversion/1 -> Mux/1
  Data Type Conversion6/1 -> Mux/7
  Data Type Conversion1/1 -> Mux/2
  Data Type Conversion5/1 -> Mux/6
  Data Type Conversion2/1 -> Mux/3
  Data Type Conversion4/1 -> Mux/5
  Data Type Conversion3/1 -> Mux/4
  CAN_TYPE1_RX_M1_C1/7 -> Data Type Conversion6/1  "byte7"
  CAN_TYPE1_RX_M1_C1/8 -> Data Type Conversion7/1  "byte8"
  CAN_TYPE1_RX_M1_C1/5 -> Data Type Conversion4/1  "byte5"
  CAN_TYPE1_RX_M1_C1/6 -> Data Type Conversion5/1  "byte6"
  CAN_TYPE1_RX_M1_C1/2 -> Data Type Conversion1/1  "byte2"
  CAN_TYPE1_RX_M1_C1/4 -> Data Type Conversion3/1  "byte4"
  CAN_TYPE1_RX_M1_C1/3 -> Data Type Conversion2/1  "byte3"
  CAN_TYPE1_RX_M1_C1/1 -> Data Type Conversion/1  "byte1"
  Bus Creator3/1 -> TPDT_FF_00/1  "TPDT_FF_00"

== system SUB_ECU_L4_MABX_HW_Interface/CAN_Truck166/CAN1_RX_TPDT_FF_00/SelectChannel ==
  In1 : Inport
  Constant : Constant  Value=ENUM_CAN_RX_T.RX_CAN_1
  Constant1 : Constant  Value=ENUM_CAN_RX_T.RX_CAN_2
  Constant2 : Constant  Value=ENUM_CAN_RX_T.RX_CAN_3
  Constant3 : Constant  Value=ENUM_CAN_RX_T.RX_CAN_4
  Constant4 : Constant  Value=ENUM_CAN_RX_T.RX_CAN_5
  Constant5 : Constant  Value=ENUM_CAN_RX_T.RX_CAN_6
  EQ{,1..5} (6 alike) : PTC_MBDS_LIB/MBDS Standard Library/Basic Operations/Logic and Bit Operations/EQ  InputSameDT=on  PTC_MBDS_BlockVersion=5.41  PTC_BlockType=PTC_MBDS_EQ
      settings: SourceProductName=PACCAR Technical Center MBDS Library
  CAN1 : Outport
  CAN2 : Outport  Port=2
  CAN3 : Outport  Port=3
  CAN4 : Outport  Port=4
  CAN5 : Outport  Port=5
  CAN6 : Outport  Port=6
  wires:
  EQ5/1 -> CAN6/1
  EQ4/1 -> CAN5/1
  EQ3/1 -> CAN4/1
  EQ2/1 -> CAN3/1
  EQ1/1 -> CAN2/1
  Constant5/1 -> EQ5/2
  Constant4/1 -> EQ4/2
  Constant3/1 -> EQ3/2
  Constant2/1 -> EQ2/2
  Constant1/1 -> EQ1/2
  EQ/1 -> CAN1/1
  Constant/1 -> EQ/2
  In1/1 -> EQ/1, EQ1/1, EQ2/1, EQ3/1, EQ4/1, EQ5/1

== system SUB_ECU_L4_MABX_HW_Interface/CAN_Truck166/CAN_RX_ACC1_2A/RX_CAN_1 ==
  Enable : Inport
  ACC1_2A_ : rtican/RTICAN Receive (RX)   Reserved1=[]  Reserved2=[]  Reserved3=[]  Reserved4=[]  SfcnMessage=[]  Msg_Struct=[]  BoardTypeNo=[]  BoardNo=[]  ChannelNo=[]  Parameters=[]  DialogFcn=[]  UnitName=[]  Revision=[]  UnitValues=[]  DSProperties=struct('RTI',struct('Version',uint32(5),'BlockType',struct('isSLSource',uint8(1),'isSLSink',uint8(1),'isHWSource',uint8(0),'isHWSink',uint8(0),'isSetup',uint8(0),'isInline',uint8(1),'isNonInline',uint8(0),'isInterrupt',uint8(0),'isChannelwise',uint8(0)),'IOBoardType','RTICAN','UnitType','MESSAGE','Identifier','RX','DialogType','MSVC','BlockSet','RTICAN','SlaveProcessor','CAN'))  RTIBlockInterface=struct('OutputPortsWidth',int32([1 1 1 1 1 1 1 1 1 1 1 1 1]),'OutputPortsActive',ones(1,13),'OutputPortsName',{{'SpeedOfForwardVehicle','DistanceToForwardVehicle','AdaptiveCruiseCtrlSetSpeed','AdaptiveCruiseCtrlMode','AdptveCruiseCtrlSetDistanceMode','RoadCurvature','ACCTargetDetected','ACCSystemShutoffWarning','ACCDistanceAlertSignal','ForwardCollisionWarning',['RX status'],['RX time'],['RX delta time']}},'OutputPortsDataType',{{'SS_DOUBLE','SS_DOUBLE','SS_DOUBLE','SS_DOUBLE','SS_DOUBLE','SS_DOUBLE','SS_DOUBLE','SS_DOUBLE','SS_DOUBLE','SS_DOUBLE','SS_DOUBLE','SS_DOUBLE','SS_DOUBLE'}},'OutputPortsLabel',{{'SpeedOfForwardVehicle','DistanceToForwardVehicle','AdaptiveCruiseCtrlSetSpeed','AdaptiveCruiseCtrlMode','AdptveCruiseCtrlSetDistanceMode','RoadCurvature','ACCTargetDetected','ACCSystemShutoffWarning','ACCDistanceAlertSignal','ForwardCollisionWarning','','',''}},'OutputPortsLabelMode','ON','InputPortsWidth',int32(0),'InputPortsActive',0,'DialogFcn','rtican_message_interface_gui','BlockDisplay',{{'','center'}},'IconTransparency','on','ParameterTunableNames',{{}},'InitLevel',3,'BlockName',struct('Token',{{'ACC1_2A'}}),'SampleTime',{{-1}},'TriggerPort',{{'none'}},'EnablePort',{{'yes'}})  RTIBlockParameters=struct('BoardTypeNo',{{1,'OFF',[]}},'BoardNo',{{1,'ON',[1 16]}},'ChannelNo',{{1,'ON',[1 2]}},'Parameters',{{struct('DataFileSupport',struct('DataFileSelectedMaster',1,'DataFileSelectedLocal',1,'DataFileName','c:\data\svn\truck1571\dbc\mabx_can1.dbc|c:\data\svn\truck1571\dbc\j1939_famosdbcwithfusion.dbc|','DataFileDate',{{{['31-Jan-2018 07:14:07']},{['31-Jan-2018 07:14:07']}}},'SelectedFile','dbc\j1939_famosdbcwithfusion.dbc'),'Options',struct('StatusSelected',1,'TimeSelected',1,'DeltaTimeSelected',1,'BytePortSelected',0,'MessageLengthSelected',0,'TriggerPort',struct('Selected',0,'TriggerType',0),'UserCoding',struct('Selected',0,'InterfaceFile','UserDecodingFile','FcnName','UserDecodeFcn','InportSelected',0,'InportWidth',1,'OutportSelected',0,'OutportWidth',1),'EnablePortSelected',1,'SignalOnPortnameSelected',1,'UseRXService',1),'Message',struct('MsgOnBlocknameSelected',1,'MsgName','ACC1_2A','MsgIdFormat',1,'MsgId',285110058,'MsgLength',8,'NumSignals',10,'SampleTime',-1,'Signal',struct('SgnName',{'SpeedOfForwardVehicle','DistanceToForwardVehicle','AdaptiveCruiseCtrlSetSpeed','AdaptiveCruiseCtrlMode','AdptveCruiseCtrlSetDistanceMode','RoadCurvature','ACCTargetDetected','ACCSystemShutoffWarning','ACCDistanceAlertSignal','ForwardCollisionWarning'},'SgnStartBit',{0,8,16,24,27,32,48,50,52,54},'SgnLength',{8,8,8,3,3,16,2,2,2,2},'SgnType',{0,0,0,0,0,0,0,0,0,0},'ModeValue',{-1,-1,-1,-1,-1,-1,-1,-1,-1,-1},'DataType',{0,0,0,0,0,0,0,0,0,0},'ByteLayout',{0,0,0,0,0,0,0,0,0,0},'Factor',{1,1,1,1,1,2^-7,1,1,1,1},'Offset',{0,0,0,0,0,-250,0,0,0,0},'SgnComment',{{['Absolute velocity of the preceding vehicle situated within 250 m in the same lane and moving in the same direction.']},{['Distance to the preceding vehicle situated within 250 m in the same lane and moving in the same direction.']},{['Value of the desired (chosen) velocity of the adaptive cruise control system.']},{['This parameter is used to indicate the current state, or mode, of operation by the Adaptive Cruise Control (ACC) device.']},{['Selected distance mode for adaptive cruise control.']},{['Estimated value of the current road curvature for use by the adaptive cruise control system.']},{['Signal to indicate to the driver that the ACC system has detected a target.']},{['Signal to warn the driver of system deactivation due to non-driver actions.']},{['Signal to indicate to the operator that the ACC system is not able to maintain the distance to the target.']},{['This parameter indicates if a collision is imminent and strong driver reaction either by braking hard or by an avoidance']}},'SgnUnit',{'km/h','m','km/h','','','1/km','','','',''},'Min',{0,0,0,0,0,-250,0,0,0,0},'Max',{250,250,250,7,7,251.992,3,3,3,3},'SLDataType',{'SS_DOUBLE','SS_DOUBLE','SS_DOUBLE','SS_DOUBLE','SS_DOUBLE','SS_DOUBLE','SS_DOUBLE','SS_DOUBLE','SS_DOUBLE','SS_DOUBLE'}),'MsgIdNumFormat',1,'MsgComment',{{['Adaptive Cruise Control']}}),'Version',1.2,'general',struct('isFromLib',0)),'OFF',[]}},'GroupId',{{struct('Group',{{'RTICAN'}},'No',1,'Behavior',{{'NAMECHANGE'}},'BlockType',{{'SINK'}},'NameChangeFlag',0),'OFF',[]}},'SFcnRTICANMessage',{{struct('MsgType','RX','SFcnPortType','Scalar','MsgName','ACC1_2A','MsgIdFormat','XTD','MsgId',285110058,'MsgLength',8,'NumSignals',10,'SampleTime',-1,'Signal',struct('SgnName',{'SpeedOfForwardVehicle','DistanceToForwardVehicle','AdaptiveCruiseCtrlSetSpeed','AdaptiveCruiseCtrlMode','AdptveCruiseCtrlSetDistanceMode','RoadCurvature','ACCTargetDetected','ACCSystemShutoffWarning','ACCDistanceAlertSignal','ForwardCollisionWarning'},'SgnStartBit',{0,8,16,24,27,32,48,50,52,54},'SgnLength',{8,8,8,3,3,16,2,2,2,2},'SgnType',{'standard','standard','standard','standard','standard','standard','standard','standard','standard','standard'},'ModeValue',{-1,-1,-1,-1,-1,-1,-1,-1,-1,-1},'DataType',{['unsigned int'],['unsigned int'],['unsigned int'],['unsigned int'],['unsigned int'],['unsigned int'],['unsigned int'],['unsigned int'],['unsigned int'],['unsigned int']},'ByteLayout',{['little endian'],['little endian'],['little endian'],['little endian'],['little endian'],['little endian'],['little endian'],['little endian'],['little endian'],['little endian']},'Factor',{1,1,1,1,1,2^-7,1,1,1,1},'Offset',{0,0,0,0,0,-250,0,0,0,0},'SLDataType',{'SS_DOUBLE','SS_DOUBLE','SS_DOUBLE','SS_DOUBLE','SS_DOUBLE','SS_DOUBLE','SS_DOUBLE','SS_DOUBLE','SS_DOUBLE','SS_DOUBLE'}),'StatusSelected','yes','TimeSelected','yes','DeltaTimeSelected','yes','BytePortSelected','no','MessageLengthSelected','no','TriggerPort',struct('Selected','no','TriggerType',0),'UserCoding',struct('Selected','no','InterfaceFile','UserDecodingFile','FcnName','UserDecodeFcn','InportSelected','no','InportWidth',1,'OutportSelected','no','OutportWidth',1),'EnablePortSelected','yes','UseRXService','yes','BoardType','DS1','BoardNo',1,'ControllerNo',1),'OFF',[]}},'TLCFileName',{{'rtican_rx_message','OFF',[]}})  RTISFcnParameters=struct('SFcnRTICANMessage','struct','TLCFileName','char')  RTIBlockParaDefault=struct('BoardTypeNo',4302,'BoardNo',1,'ChannelNo',1,'Parameters',struct('DataFileSupport',struct('DataFileSelectedMaster',0,'DataFileSelectedLocal',0,'DataFileName','','DataFileDate','','SelectedFile',['<no file selected>']),'Options',struct('StatusSelected',1,'TimeSelected',1,'DeltaTimeSelected',1,'BytePortSelected',0,'MessageLengthSelected',0,'TriggerPort',struct('Selected',0,'TriggerType','rising'),'UserCoding',struct('Selected',0,'InterfaceFile','UserDecodingFile','FcnName','UserDecodeFcn','InportSelected',0,'InportWidth',1,'OutportSelected',0,'OutportWidth',1),'EnablePortSelected',0,'SignalOnPortnameSelected',1,'UseRXService',0),'Message',struct('MsgOnBlocknameSelected',0,'MsgName',['RX Message'],'MsgIdFormat',0,'MsgId',100,'MsgLength',8,'NumSignals',1,'SampleTime',-1,'Signal',struct('SgnName',['RX signal'],'SgnStartBit',0,'SgnLength',8,'SgnType',0,'ModeValue',-1,'DataType',0,'SLDataType','SS_DOUBLE','ByteLayout',0,'Factor',1,'Offset',0,'Min',0,'Max',255,'SgnComment',{{}},'SgnUnit',''),'MsgIdNumFormat',0,'MsgComment',{{''}}),'Version',1.2,'general',struct('isFromLib',1)),'GroupId',struct('Group',{{'RTICAN'}},'No',1,'Behavior',{{'NAMECHANGE'}},'BlockType',{{'SINK'}},'NameChangeFlag',0),'SFcnRTICANMessage',struct('MsgType','RX','MsgName',['RX Message'],'MsgIdFormat','STD','MsgId',100,'MsgLength',8,'NumSignals',1,'SampleTime',-1,'Signal',struct('SgnName',['RX signal'],'SgnStartBit',0,'SgnLength',8,'SgnType','standard','ModeValue',-1,'DataType',['unsigned int'],'ByteLayout',['little endian'],'SLDataType','SS_DOUBLE','Factor',1,'Offset',0),'StatusSelected','yes','TimeSelected','yes','DeltaTimeSelected','yes','BytePortSelected','no','MessageLengthSelected','no','EnablePortSelected','no','UserCoding',struct('Selected','no','InterfaceFile','UserDecodingFile','FcnName','UserDecodeFcn','InportSelected','no','InportWidth',1,'OutportSelected','no','OutportWidth',1),'TriggerPort',struct('Selected','no','TriggerType','rising'),'UseRXService','no','BoardType','DS4302','BoardNo',1,'ControllerNo',1,'SFcnPortType','Scalar'),'TLCFileName','rtican_rx_message')
      settings: AttributesFormatString=Group Id: RTICAN1\n  SourceProductName=dSPACE RTI CAN Blockset
  Bus Creator : BusCreator  Inputs=13
  Data Type Conversion{1..7,9..13} (12 alike) : DataTypeConversion  OutDataTypeStr=double  SaturateOnIntegerOverflow=on
  Data Type Conversion8 : DataTypeConversion  OutDataTypeStr=boolean  SaturateOnIntegerOverflow=on
  ACC1_2A : Outport
  wires:
  Data Type Conversion2/1 -> Bus Creator/2  "DistanceToForwardVehicle"
  Data Type Conversion1/1 -> Bus Creator/1  "SpeedOfForwardVehicle"
  Data Type Conversion3/1 -> Bus Creator/3  "AdaptiveCruiseCtrlSetSpeed"
  Data Type Conversion4/1 -> Bus Creator/4  "AdaptiveCruiseCtrlMode"
  Data Type Conversion5/1 -> Bus Creator/5  "AdptveCruiseCtrlSetDistanceMode"
  Data Type Conversion6/1 -> Bus Creator/6  "RoadCurvature"
  Data Type Conversion7/1 -> Bus Creator/7  "ACCTargetDetected"
  Data Type Conversion11/1 -> Bus Creator/8  "ACCSystemShutoffWarning"
  Data Type Conversion12/1 -> Bus Creator/9  "ACCDistanceAlertSignal"
  Data Type Conversion13/1 -> Bus Creator/10  "ForwardCollisionWarning"
  ACC1_2A_/2 -> Data Type Conversion2/1  "DistanceToForwardVehicle"
  ACC1_2A_/1 -> Data Type Conversion1/1  "SpeedOfForwardVehicle"
  ACC1_2A_/3 -> Data Type Conversion3/1  "AdaptiveCruiseCtrlSetSpeed"
  ACC1_2A_/4 -> Data Type Conversion4/1  "AdaptiveCruiseCtrlMode"
  ACC1_2A_/5 -> Data Type Conversion5/1  "AdptveCruiseCtrlSetDistanceMode"
  ACC1_2A_/6 -> Data Type Conversion6/1  "RoadCurvature"
  ACC1_2A_/7 -> Data Type Conversion7/1  "ACCTargetDetected"
  ACC1_2A_/8 -> Data Type Conversion11/1  "ACCSystemShutoffWarning"
  ACC1_2A_/9 -> Data Type Conversion12/1  "ACCDistanceAlertSignal"
  ACC1_2A_/10 -> Data Type Conversion13/1  "ForwardCollisionWarning"
  Bus Creator/1 -> ACC1_2A/1  "ACC1_2A"
  Enable/1 -> ACC1_2A_/Enable
  ACC1_2A_/13 -> Data Type Conversion10/1
  ACC1_2A_/12 -> Data Type Conversion9/1
  ACC1_2A_/11 -> Data Type Conversion8/1
  Data Type Conversion8/1 -> Bus Creator/11  "RX_status"
  Data Type Conversion9/1 -> Bus Creator/12  "RX_time"
  Data Type Conversion10/1 -> Bus Creator/13  "RX_delta_time"
